simulink model "multiple_EL_2018a"  (R2018a)
settings: Solver=ode4  StartTime=0.0  StopTime=20  FixedStep=0.001  RelTol=1e-3  EnableMultiTasking=on
settings Model: ExtModeTrigMode=oneshot  ExtModeArmWhenConnect=off  Creator=hp  LastModifiedBy=Administrator
settings DataIOCC: SaveFormat=Array  SignalLoggingSaveFormat=ModelDataLogs  SignalLoggingName=sigsOut
settings OptimizationCC: BooleanDataType=off  ExpressionDepthLimit=2147483647  InitFltsAndDblsToZero=on  LifeSpan=inf
settings DebuggingCC: SaveWithParameterizedLinksMsg=none  UnderspecifiedInitializationDetection=Classic  MergeDetectMultiDrivingBlocksExec=none  SignalResolutionControl=TryResolveAllWithWarning  MultiTaskDSMMsg=warning  MultiTaskCondExecSysMsg=none  FcnCallInpInsideContextMsg=warning  StateNameClashWarn=warning  LibraryContextMissingDiagnostic=warning  SFUnexpectedBacktrackingDiag=warning  SFNoUnconditionalDefaultTransitionDiag=warning  SFExecutionAtInitializationDiag=none
settings HardwareCC: ProdBitPerPointer=32  ProdBitPerSizeT=32  ProdBitPerPtrDiffT=32  ProdLargestAtomicFloat=None  ProdIntDivRoundTo=Undefined  ProdEndianess=Unspecified  ProdWordSize=32  ProdHWDeviceType=32-bit Generic  TargetUnknown=on
settings ModelReferenceCC: PropagateSignalLabelsOutOfModel=off
settings CodeAppCC: StateflowObjectComments=on
settings GRTTargetCC: TargetFcnLib=ansi_tfl_tmw.mat  TargetLangStandard=C89/C90 (ANSI)  GeneratePreprocessorConditionals=Disable all  CombineOutputUpdateFcns=off  GRTInterface=on
settings ConfigComp: CovMetricSettings=dw  CovHtmlReporting=on  CovSaveCumulativeToWorkspaceVar=on  CovSaveSingleToWorkspaceVar=on  CovExternalEMLEnable=off

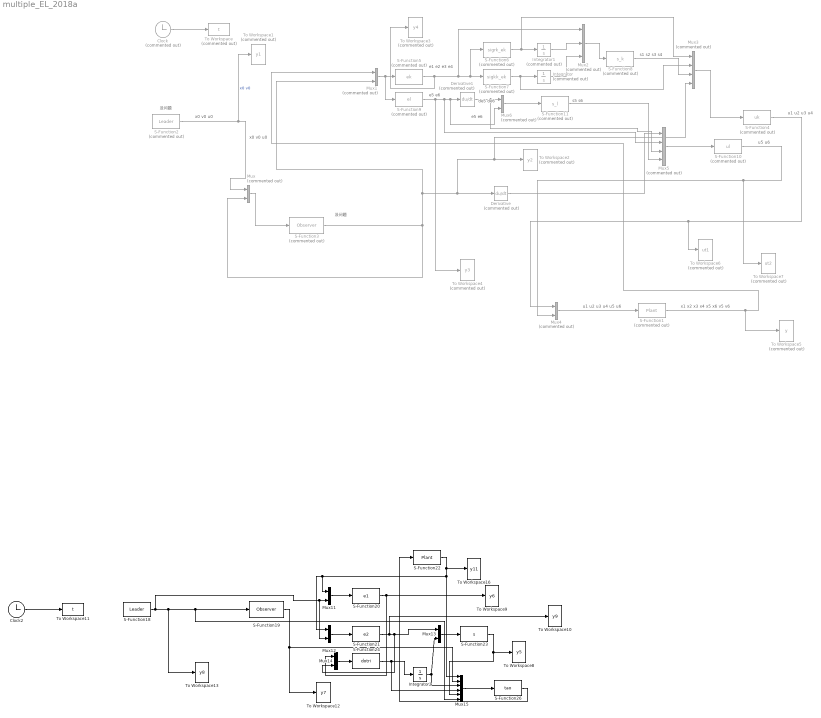
== system multiple_EL_2018a ==
  note: s5 s6
  note: s1 s2 s3 s4
  note: de5 de6
  note: e1 e2 e3 e4
  note: e5 e6
  note: u1 u2 u3 u4 u5 u6
  note: u1 u2 u3 u4
  note: x1 x2 x3 x4 x5 x6 v5 v6
  note: x0 v0 u0
  note: 没问题
  note: 没问题
  note: x0 v0 u0
  note: u5 u6
  note: e5 e6
  Clock : Clock  Commented=on
  Clock2 : Clock
  Derivative : Derivative  Commented=on
  Derivative1 : Derivative  Commented=on
  Integrator : Integrator  Commented=on
  Integrator1 : Integrator  Commented=on
  Integrator2 : Integrator
  Mux{,1,4,6} (4 alike) : Mux  Commented=on  Inputs=2
  Mux{11..14} (4 alike) : Mux  Inputs=2
  Mux15 : Mux  Inputs=6
  Mux2 : Mux  Commented=on  Inputs=3
  Mux3 : Mux  Commented=on
  Mux5 : Mux  Commented=on
  S-Function1 : S-Function  Commented=on  FunctionName=Plant  SFunctionDeploymentMode=off  EnableBusSupport=off
  S-Function10 : S-Function  Commented=on  FunctionName=ul  SFunctionDeploymentMode=off  EnableBusSupport=off
  S-Function11 : S-Function  Commented=on  FunctionName=s_l  SFunctionDeploymentMode=off  EnableBusSupport=off
  S-Function18 : S-Function  FunctionName=Leader  SFunctionDeploymentMode=off  EnableBusSupport=off
  S-Function19 : S-Function  FunctionName=Observer  SFunctionDeploymentMode=off  EnableBusSupport=off
  S-Function2 : S-Function  Commented=on  FunctionName=Leader  SFunctionDeploymentMode=off  EnableBusSupport=off
  S-Function20 : S-Function  FunctionName=e1  SFunctionDeploymentMode=off  EnableBusSupport=off
  S-Function21 : S-Function  FunctionName=e2  SFunctionDeploymentMode=off  EnableBusSupport=off
  S-Function22 : S-Function  FunctionName=Plant  SFunctionDeploymentMode=off  EnableBusSupport=off
  S-Function23 : S-Function  FunctionName=s  SFunctionDeploymentMode=off  EnableBusSupport=off
  S-Function24 : S-Function  FunctionName=dotri  SFunctionDeploymentMode=off  EnableBusSupport=off
  S-Function26 : S-Function  FunctionName=tao  SFunctionDeploymentMode=off  EnableBusSupport=off
  S-Function3 : S-Function  Commented=on  FunctionName=Observer  SFunctionDeploymentMode=off  EnableBusSupport=off
  S-Function4 : S-Function  Commented=on  FunctionName=uk  SFunctionDeploymentMode=off  EnableBusSupport=off
  S-Function5 : S-Function  Commented=on  FunctionName=ek  SFunctionDeploymentMode=off  EnableBusSupport=off
  S-Function6 : S-Function  Commented=on  FunctionName=sigrk_ek  SFunctionDeploymentMode=off  EnableBusSupport=off
  S-Function7 : S-Function  Commented=on  FunctionName=sigkk_ek  SFunctionDeploymentMode=off  EnableBusSupport=off
  S-Function8 : S-Function  Commented=on  FunctionName=s_k  SFunctionDeploymentMode=off  EnableBusSupport=off
  S-Function9 : S-Function  Commented=on  FunctionName=el  SFunctionDeploymentMode=off  EnableBusSupport=off
  To Workspace : ToWorkspace  Commented=on  VariableName=t  SampleTime=-1
  To Workspace1 : ToWorkspace  Commented=on  VariableName=y1  SampleTime=-1
  To Workspace10 : ToWorkspace  VariableName=y9  SampleTime=-1
  To Workspace11 : ToWorkspace  VariableName=t  SampleTime=-1
  To Workspace12 : ToWorkspace  VariableName=y7  SampleTime=-1
  To Workspace13 : ToWorkspace  VariableName=y8  SampleTime=-1
  To Workspace16 : ToWorkspace  VariableName=y11  SampleTime=-1
  To Workspace2 : ToWorkspace  Commented=on  VariableName=y2  SampleTime=-1
  To Workspace3 : ToWorkspace  Commented=on  VariableName=y4  SampleTime=-1
  To Workspace4 : ToWorkspace  Commented=on  VariableName=y3  SampleTime=-1
  To Workspace5 : ToWorkspace  Commented=on  VariableName=y  SampleTime=-1
  To Workspace6 : ToWorkspace  Commented=on  VariableName=ut1  SampleTime=-1
  To Workspace7 : ToWorkspace  Commented=on  VariableName=ut2  SampleTime=-1
  To Workspace8 : ToWorkspace  VariableName=y5  SampleTime=-1
  To Workspace9 : ToWorkspace  VariableName=y6  SampleTime=-1
  wires:
  Clock/1 -> To Workspace/1
  S-Function2/1 -> Mux/1, To Workspace1/1  "x0 v0"
  Mux/1 -> S-Function3/1
  S-Function3/1 -> Mux3/4, To Workspace2/1, Derivative/1, Mux1/2, Mux/2
  Mux1/1 -> S-Function9/1, S-Function5/1
  S-Function1/1 -> To Workspace5/1, Mux1/1
  S-Function5/1 -> To Workspace3/1, Mux2/1, S-Function7/1, S-Function6/1
  S-Function7/1 -> Mux3/2, Integrator/1
  S-Function6/1 -> Mux3/1, Integrator1/1
  Mux2/1 -> S-Function8/1
  Integrator1/1 -> Mux2/2
  S-Function8/1 -> Mux3/3
  Mux3/1 -> S-Function4/1
  Mux4/1 -> S-Function1/1
  S-Function4/1 -> To Workspace6/1, Mux4/1
  S-Function10/1 -> To Workspace7/1, Mux4/2
  S-Function9/1 -> To Workspace4/1, Mux5/2, Mux6/2, Derivative1/1
  Derivative1/1 -> Mux6/1, Mux5/3
  Mux6/1 -> S-Function11/1
  Derivative/1 -> Mux5/1
  S-Function11/1 -> Mux5/4
  Mux5/1 -> S-Function10/1
  Integrator/1 -> Mux2/3
  Clock2/1 -> To Workspace11/1
  S-Function18/1 -> Mux12/2, Mux11/2, Mux15/6, S-Function19/1, To Workspace13/1
  S-Function19/1 -> Mux15/2, To Workspace12/1
  Mux11/1 -> S-Function20/1
  Mux12/1 -> S-Function21/1
  S-Function22/1 -> To Workspace16/1, Mux15/1, Mux11/1, Mux12/1
  Mux13/1 -> S-Function23/1
  S-Function21/1 -> To Workspace10/1, Mux14/2, Mux13/1
  Mux14/1 -> S-Function24/1
  S-Function20/1 -> Mux14/1, To Workspace9/1
  S-Function24/1 -> Mux15/4, Integrator2/1
  Integrator2/1 -> Mux15/3, Mux13/2
  Mux15/1 -> S-Function26/1
  S-Function26/1 -> S-Function22/1
  S-Function23/1 -> To Workspace8/1, Mux15/5
